simulink model "MotorDriveUnit_TestModel"  (R2025a)
settings: Solver=daessc  StartTime=0.0  StopTime=400  RelTol=1e-3
PreLoadFcn:
  | MotorDriveUnit_TestModelSetup
undefined symbols (not defined in the file or in its folder): batteryHV, Minus, Plus
libraries: fl_lib x22, nesl_utility x10, simulink x5, sdl_lib x1
settings Model: Creator=isaacito  LastModifiedBy=isaacito
settings DataIOCC: DSMLogging=off
settings OptimizationCC: ReuseModelBlockBuffer=off
settings ModelReferenceCC: EnableRefExpFcnMdlSchedulingChecks=on
settings RTWCC: GPUComputeCapability=3.5
settings SimscapeCC: SimscapeLogType=all  SimscapeLogSimulationStatistics=on  SimscapeLogLimitData=off

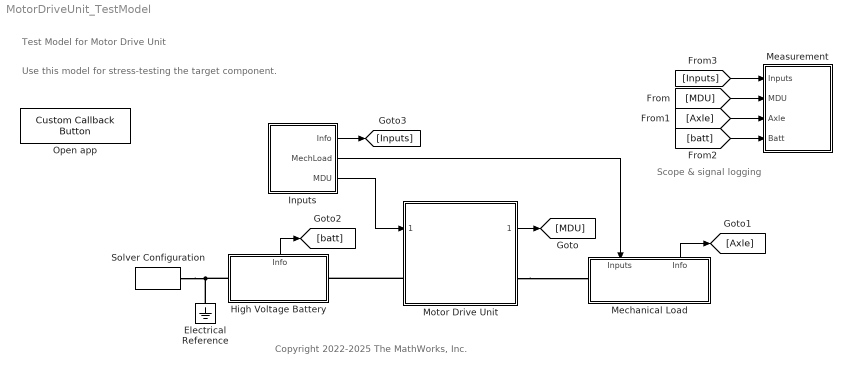
== system MotorDriveUnit_TestModel ==
  note: Test Model for Motor Drive Unit
  note: Copyright 2022-2025 The MathWorks, Inc.
  note: Use this model for stress-testing the target component.
  note: Scope & signal logging
  Electrical Reference : fl_lib/Electrical/Electrical Elements/Electrical Reference
  High Voltage Battery : Subsystem
      settings: PortSchema="{\"entries\":[{\"content\":{\"sides\":[{\"content\":{\"connectorIds\":[\"LConn1\"]},\"type\":\"ConnectorPlacement.EquallySpacedRectSide\",\"uuid\":\"8acd7e9a-bb08-4de6-aa14-0989ebba81b9\"},{\"content\":{\"connectorIds\":[\"RConn1\"],\"side\":\"RIGHT\"},\"type\":\"ConnectorPlacement.EquallySpacedRectSide\",\"uuid\":\"f80e1afc-966f-4d6b-84f9-f0b60dd6f20c\"},{\"content\":{\"connectorIds\":[\"Out1\"],\"side\":\"TOP\"},\"type\":\"ConnectorPlacement.EquallySpacedRectSide\",\"uuid\":\"52ccb2b1-bd5e-4dcb-b9b6-0ef03b912c33\"}]},\"type\":\"ConnectorPlacement.EquallySpacedConnector\",\"uuid\":\"b55f48a4-f283-4a77-8513-99b31abb285a\"}],\"packageUris\":[\"http://schema.mathworks.com/mf0/Connector/R2020b\"],\"version\":\"1.0\"}"
  Inputs : Subsystem
  Measurement : Subsystem
  Mechanical Load : Subsystem
      settings: PortSchema="{\"entries\":[{\"content\":{\"sides\":[{\"content\":{\"connectorIds\":[\"LConn1\"]},\"type\":\"ConnectorPlacement.EquallySpacedRectSide\",\"uuid\":\"18221845-08ef-4cf2-b090-320221152030\"},{\"content\":{\"connectorIds\":[],\"side\":\"RIGHT\"},\"type\":\"ConnectorPlacement.EquallySpacedRectSide\",\"uuid\":\"d5b0548b-74c8-455a-9783-7dc299f3571f\"},{\"content\":{\"connectorIds\":[\"In1\",\"Out1\"],\"side\":\"TOP\"},\"type\":\"ConnectorPlacement.EquallySpacedRectSide\",\"uuid\":\"542d8e55-6d7f-4c9a-9fdc-66897ed9f466\"}]},\"type\":\"ConnectorPlacement.EquallySpacedConnector\",\"uuid\":\"3cd4c536-0337-4305-a842-969bfb1fefe3\"}],\"packageUris\":[\"http://schema.mathworks.com/mf0/Connector/R2020b\"],\"version\":\"1.0\"}"
  Motor Drive Unit : Subsystem  ReferencedSubsystem=MotorDriveUnit_Basic_refsub
      settings: OpenFcn=|
      | % Look under mask:
      | open_system(gcb, "force")
  Open app : CustomCallbackButton  Configuration="{\"components\":[{\"name\":\"BackgroundImageComponent\",\"settings\":{\"image\":{\"size\":[0,0],\"src\":\"default\",\"srcOrientation\":\"Right\"},\"position\":[0,0,1,1]}},{\"name\":\"ButtonStateComponent\",\"settings\":{\"buttonType\":\"momentary\",\"clickFcn\":\"MotorDriveUnitApp\\n\",\"onValue\":1,\"position\":[0,0,1,1],\"pressDelay\":\"500\",\"pressFcn\":\"\",\"repeatInterval\":\"0\",\"states\":[{\"horizontalAlignment\":\"center\",\"image\":{\"position\":[0,0,1,1],\"size\":[1,1],\"src\":\"default\",\"srcOrientation\":\"Right\"},\"label\":{\"color\":[0.01176470588,0.01176470588,0.01176470588,1],\"icon\":{\"size\":[0,0],\"src\":\"default\",\"srcOrientation\":\"Right\"},\"iconOffset\":0,\"iconPlacement\":\"left\",\"opacity\":1,\"show\":true,\"text\":{\"content\":\"Open app\",\"font\":\"Helvetica\"}},\"labelOffset\":[0,0],\"verticalAlignment\":\"middle\"},{\"horizontalAlignment\":\"center\",\"image\":{\"position\":[0,0,1,1],\"size\":[1,1],\"src\":\"default\",\"srcOrientation\":\"Right\"},\"label\":{\"color\":[0.01176470588,0.01176470588,0.01176470588,1],\"icon\":{\"size\":[0,0],\"src\":\"default\",\"srcOrientation\":\"Right\"},\"iconOffset\":0,\"iconPlacement\":\"left\",\"opacity\":1,\"show\":true,\"text\":{\"content\":\"Open app\",\"font\":\"Helvetica\"}},\"labelOffset\":[0,0],\"verticalAlignment\":\"middle\"},{\"horizontalAlignment\":\"center\",\"image\":{\"position\":[0,0,1,1],\"size\":[1,1],\"src\":\"default\",\"srcOrientation\":\"Right\"},\"label\":{\"color\":[0.01176470588,0.01176470588,0.01176470588,1],\"icon\":{\"size\":[0,0],\"src\":\"default\",\"srcOrientation\":\"Right\"},\"iconOffset\":0,\"iconPlacement\":\"left\",\"opacity\":1,\"show\":true,\"text\":{\"content\":\"Open app\",\"font\":\"Helvetica\"}},\"labelOffset\":[0,0],\"verticalAlignment\":\"middle\"},{\"horizontalAlignment\":\"center\",\"image\":{\"position\":[0,0,1,1],\"size\":[1,1],\"src\":\"default\",\"srcOrientation\":\"Right\"},\"label\":{\"color\":[0.01176470588,0.01176470588,0.01176470588,1],\"icon\":{\"size\":[0,0],\"src\":\"default\",\"srcOrientation\":\"Right\"},\"iconOffset\":0,\"iconPlacement\":\"left\",\"opacity\":1,\"show\":true,\"text\":{\"content\":\"Open app\",\"font\":\"Helvetica\"}},\"labelOffset\":[0,0],\"verticalAlignment\":\"middle\"}]}},{\"name\":\"ForegroundImageComponent\",\"settings\":{\"image\":{\"size\":[0,0],\"src\":\"default\",\"srcOrientation\":\"Right\"},\"isForeground\":1,\"position\":[0,0,1,1]}}],\"derived\":{\"blockParameters\":{\"AutoActivate\":true,\"ButtonText\":\"Open app\",\"ButtonType\":\"Momentary\",\"ClickFcn\":\"MotorDriveUnitApp\\n\",\"OnValue\":1,\"PressDelay\":\"500\",\"PressFcn\":\"\",\"RepeatInterval\":\"0\",\"fixedAspectRatio\":\"on\"}},\"settings\":{\"BindingType\":\"standalone\",\"autoActivate\":true,\"backgroundColor\":[244,244,244,1],\"backgroundOffset\":0.2,\"backgroundOpacity\":1,\"fixedAspectRatio\":\"on\",\"foregroundColor\":[0.01176470588,0.01176470588,0.01176470588,1],\"migratedFromLegacy\":true,\"useBackgroundColor\":true,\"variant\":\"callback\",\"version\":\"R2025a\"},\"type\":\"Button\"}"  CustomBackgroundColor="{\"color\":[0.9568627451,0.9568627451,0.9568627451],\"show\":true}"
  Solver Configuration : nesl_utility/Solver Configuration  PhysicalDomain=network_engine_domain  SubClassName=solver  LeftPortType=input  RightPortType=generic  Tones=[]  Harmonics=[]  SimulateNoise=off  Profile=off  UseLocalSampling=off  EnableSwitchedLinearOptims=on  FrequencyDomain=off  UseCCode=off  RelTol=0.001  AbsTol=1e-06  MinStep=1e-09  ToWorkspace=off  RevertToSquareIcSolve=off  NumHomotopyIterations=100  PhasorMode=off  PhasorModeNumHarmonics=1  ConsistencySolver=NEWTON_FTOL  IndexReductionMethod=DerivativeReplacement  DoDC=off  ResidualTolerance=1e-09  ConsistencyTolSource=GLOBAL  ConsistencyAbsTol=0.001  ConsistencyRelTol=0.001  ConsistencyTolFactor=0.001  UseLocalSolver=off  LocalSolverChoice=NE_BACKWARD_EULER_ADVANCER  ResolveIndetEquations=on  FunctionEvalNumThread=1  LocalSolverSampleTime=0.001  DoFixedCost=off  MaxNonlinIter=3  MaxModeIter=2  ComputeImpulses=off  ImpulseIterations=2  LinearAlgebra=auto  LinearAlgebraNumThread=0  EquationFormulation=NE_TIME_EF  DelaysMemoryBudget=1024  AutomaticFiltering=on  FilteringTimeConstant=0.001  PartitionStorageMethod=AS_NEEDED  PartitionMemoryBudget=1024  PartitionMethod=ROBUST  MultibodyUseLocalSolver=off  MultibodyLocalSolverChoice=ODE1  MultibodyLocalSolverSampleTime=0.001
      settings: AttributesFormatString=Local solver %<UseLocalSolver>
  wires:
  Motor Drive Unit/1 -> [MDU]
  [MDU] -> Measurement/2(MDU)
  Inputs/3(MDU) -> Motor Drive Unit/1
  [Axle] -> Measurement/3(Axle)
  High Voltage Battery/1(Info) -> [batt]
  [batt] -> Measurement/4(Batt)
  Inputs/2(MechLoad) -> Mechanical Load/1(Inputs)
  Mechanical Load/1(Info) -> [Axle]
  Inputs/1(Info) -> [Inputs]
  [Inputs] -> Measurement/1(Inputs)
  connections:
  Motor Drive Unit/LConn1 -- High Voltage Battery/RConn1
  Electrical Reference/LConn1 -- High Voltage Battery/LConn1 -- Solver Configuration/RConn1
  Motor Drive Unit/RConn1 -- Mechanical Load/LConn1

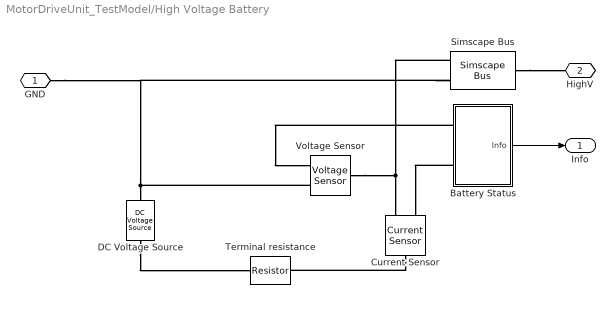
== system MotorDriveUnit_TestModel/High Voltage Battery ==
  Battery Status : Subsystem
  Current Sensor : fl_lib/Electrical/Electrical Sensors/Current Sensor
  DC Voltage Source : fl_lib/Electrical/Electrical Sources/DC Voltage Source  v0=batteryHV.nominalVoltage_V V
      settings: AttributesFormatString=%<v0> [%<v0_unit>]
  Simscape Bus : SimscapeBus  HierarchyStrings=Plus;Minus  ConnectionType=Bus: Bus_HighVoltage
      settings: AttributesFormatString=%<ConnectionType>
  Terminal resistance : fl_lib/Electrical/Electrical Elements/Resistor  R=batteryHV.internalResistance_Ohm Ohm  i_specify=off  i_priority=High  i=0 A  i_nominal_specify=off  i_nominal_value=1  i_nominal_unit=A  v_specify=off  v_priority=High  v=0 V  v_nominal_specify=off  v_nominal_value=1  v_nominal_unit=V
      settings: AttributesFormatString=%<R> [%<R_unit>]
  Voltage Sensor : fl_lib/Electrical/Electrical Sensors/Voltage Sensor
  GND : PMIOPort  Side=Left
  HighV : PMIOPort  Port=2  Side=Right
  Info : Outport
  wires:
  Battery Status/1(Info) -> Info/1
  connections:
  DC Voltage Source/RConn1 -- Simscape Bus/LConn2 -- GND/RConn1 -- Voltage Sensor/RConn2
  Simscape Bus/LConn1 -- Voltage Sensor/LConn1 -- Current Sensor/RConn2
  Battery Status/LConn2 -- Current Sensor/RConn1
  Simscape Bus/RConn1 -- HighV/RConn1
  Current Sensor/LConn1 -- Terminal resistance/RConn1
  DC Voltage Source/LConn1 -- Terminal resistance/LConn1
  Battery Status/LConn1 -- Voltage Sensor/RConn1

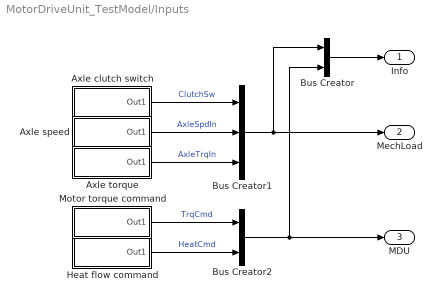
== system MotorDriveUnit_TestModel/Inputs ==
  Axle clutch switch : Subsystem  mask(Piece-Wise Constant Signal){dataPoints=[0 0;1 0]}
      mask prompts: dataPoints "Data points"
      mask help:
      | This block generates a piece-wise constant signal. Data points parameter takes an N-by-2 matrix where each row specifies a constant segment. First column defines the start time of constant segment, and second column specifies the value of it. The value continues until the value of the next segment is defined. The values of the two consecutive rows are connected with a discrete jump.
      |
      | For example, a matrix [0 6; 1 7;2 5] for Data points defines a signal as follows. First row defines a constant segment from t=0 of value 6. Second row defines a point at t=1 of value 7. Third row defines a constant segment from t=2 of value 5. The value makes a discrete jump from one segment to the next.
      mask init:
      | sig = SignalDesigner("PieceWiseConstant");
      | 
      | % Initialization function can access parameter names directly
      | sig.XYData = dataPoints;
      | 
      | update(sig)
      | 
      | SignalSourceBlockCallback.setDataToLookupTableBlock( ...
      |   SignalObject = sig, ...
      |   PathToBlock = [gcb '/1-D Lookup Table']);
      mask DialogControl Control3 Prompt: invisible horizontal spacer 1
      mask DialogControl Control4 Prompt: invisible horizontal spacer 2
      mask DialogControl Control5 Prompt: invisible horizontal spacer 3
      mask DialogControl PlotButton Prompt: Plot
      mask DialogControl PlotButton Callback: SignalSourceBlockCallback.plotPieceWiseConstant(gcb)
      mask Display: disp("Piece-Wise" + newline + "Constant")
  Axle speed : Subsystem  mask(Continuous Multi-Step Signal){dataPoints=[0 1 0], deltaT=10}
      mask prompts: dataPoints "Data points"; deltaT "Interpolation step [s]"
      mask help:
      | This block generates a signal consisting of smoothly connected flat segments. Data points parameter takes an N-by-3 matrix where each row specifies a flat segment. First column and second column define start and end time of the segment, respectively. Third column defines the value of the segment. Second column can also be NaN to define a point value. Flat segments and point values are smoothly interpolated by Akima spline with the specified interpolation step.
      |
      | For example, a matrix [0 1 5; 3 nan 9; 6 8 7] for Data points defines a signal as follows. First row defines a flat segment from t=0 to t=1 of value 5. Second row defines a point at t=3 of value 9. Third row defines a flat segment from t=6 to t=8 of value 7.
      mask init:
      | sig = SignalDesigner("ContinuousMultiStep");
      | 
      | % Initialization function can access parameter names directly
      | sig.XYData = dataPoints;
      | sig.DeltaX = deltaT;
      | 
      | update(sig)
      | 
      | SignalSourceBlockCallback.setDataToLookupTableBlock( ...
      |   SignalObject = sig, ...
      |   PathToBlock = [gcb '/1-D Lookup Table']);
      mask DialogControl Control3 Prompt: horizontal spacer 1
      mask DialogControl Control4 Prompt: horizontal spacer 2
      mask DialogControl Control5 Prompt: horizontal spacer 3
      mask DialogControl PlotButton Prompt: Plot
      mask DialogControl PlotButton Callback: SignalSourceBlockCallback.plotContinuousMultiStep(gcb);
      mask Display: disp("Continuous" + newline + "Multi-Step")
  Axle torque : Subsystem  mask(Continuous Multi-Step Signal){dataPoints=[0 20 0;21 300 -10], deltaT=0.1}
      mask prompts: dataPoints "Data points"; deltaT "Interpolation step [s]"
      mask help:
      | This block generates a signal consisting of smoothly connected flat segments. Data points parameter takes an N-by-3 matrix where each row specifies a flat segment. First column and second column define start and end time of the segment, respectively. Third column defines the value of the segment. Second column can also be NaN to define a point value. Flat segments and point values are smoothly interpolated by Akima spline with the specified interpolation step.
      |
      | For example, a matrix [0 1 5; 3 nan 9; 6 8 7] for Data points defines a signal as follows. First row defines a flat segment from t=0 to t=1 of value 5. Second row defines a point at t=3 of value 9. Third row defines a flat segment from t=6 to t=8 of value 7.
      mask init: same as MotorDriveUnit_TestModel/Inputs/Axle speed
      mask DialogControl Control3 Prompt: horizontal spacer 1
      mask DialogControl Control4 Prompt: horizontal spacer 2
      mask DialogControl Control5 Prompt: horizontal spacer 3
      mask DialogControl PlotButton Prompt: Plot
      mask DialogControl PlotButton Callback: SignalSourceBlockCallback.plotContinuousMultiStep(gcb);
      mask Display: disp("Continuous" + newline + "Multi-Step")
  Bus Creator : BusCreator  Inputs=2
  Bus Creator1 : BusCreator  Inputs=3
  Bus Creator2 : BusCreator  Inputs=2
  Heat flow command : Subsystem  mask(Continuous Multi-Step Signal){dataPoints=[0 50 0;60 200 -2000;250 300 -12000], deltaT=1}
      mask prompts: dataPoints "Data points"; deltaT "Interpolation step [s]"
      mask help:
      | This block generates a signal consisting of smoothly connected flat segments. Data points parameter takes an N-by-3 matrix where each row specifies a flat segment. First column and second column define start and end time of the segment, respectively. Third column defines the value of the segment. Second column can also be NaN to define a point value. Flat segments and point values are smoothly interpolated by Akima spline with the specified interpolation step.
      |
      | For example, a matrix [0 1 5; 3 nan 9; 6 8 7] for Data points defines a signal as follows. First row defines a flat segment from t=0 to t=1 of value 5. Second row defines a point at t=3 of value 9. Third row defines a flat segment from t=6 to t=8 of value 7.
      mask init: same as MotorDriveUnit_TestModel/Inputs/Axle speed
      mask DialogControl Control3 Prompt: horizontal spacer 1
      mask DialogControl Control4 Prompt: horizontal spacer 2
      mask DialogControl Control5 Prompt: horizontal spacer 3
      mask DialogControl PlotButton Prompt: Plot
      mask DialogControl PlotButton Callback: SignalSourceBlockCallback.plotContinuousMultiStep(gcb);
      mask Display: disp("Continuous" + newline + "Multi-Step")
  Motor torque command : Subsystem  mask(Continuous Multi-Step Signal){dataPoints=[0 10 0;60 100 -300;105 200 200;205 300 250], deltaT=0.5}
      mask prompts: dataPoints "Data points"; deltaT "Interpolation step [s]"
      mask help:
      | This block generates a signal consisting of smoothly connected flat segments. Data points parameter takes an N-by-3 matrix where each row specifies a flat segment. First column and second column define start and end time of the segment, respectively. Third column defines the value of the segment. Second column can also be NaN to define a point value. Flat segments and point values are smoothly interpolated by Akima spline with the specified interpolation step.
      |
      | For example, a matrix [0 1 5; 3 nan 9; 6 8 7] for Data points defines a signal as follows. First row defines a flat segment from t=0 to t=1 of value 5. Second row defines a point at t=3 of value 9. Third row defines a flat segment from t=6 to t=8 of value 7.
      mask init: same as MotorDriveUnit_TestModel/Inputs/Axle speed
      mask DialogControl Control3 Prompt: horizontal spacer 1
      mask DialogControl Control4 Prompt: horizontal spacer 2
      mask DialogControl Control5 Prompt: horizontal spacer 3
      mask DialogControl PlotButton Prompt: Plot
      mask DialogControl PlotButton Callback: SignalSourceBlockCallback.plotContinuousMultiStep(gcb);
      mask Display: disp("Continuous" + newline + "Multi-Step")
  Info : Outport
  MechLoad : Outport  Port=2
  MDU : Outport  Port=3
  wires:
  Bus Creator/1 -> Info/1
  Motor torque command/1(Out1) -> Bus Creator2/1  "TrqCmd"
  Axle torque/1(Out1) -> Bus Creator1/3  "AxleTrqIn"
  Axle speed/1(Out1) -> Bus Creator1/2  "AxleSpdIn"
  Axle clutch switch/1(Out1) -> Bus Creator1/1  "ClutchSw"
  Bus Creator1/1 -> Bus Creator/1, MechLoad/1
  Bus Creator2/1 -> Bus Creator/2, MDU/1
  Heat flow command/1(Out1) -> Bus Creator2/2  "HeatCmd"

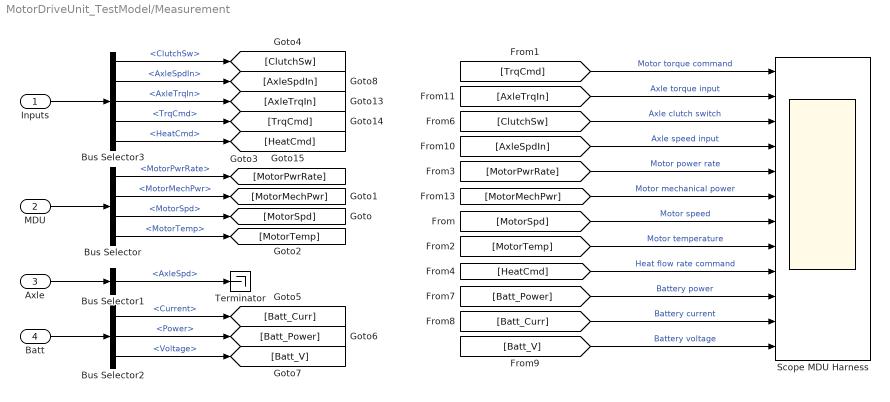
== system MotorDriveUnit_TestModel/Measurement ==
  Inputs : Inport
  MDU : Inport  Port=2
  Axle : Inport  Port=3
  Batt : Inport  Port=4
  Bus Selector : BusSelector  OutputSignals=MotorPwrRate,MotorMechPwr,MotorSpd,MotorTemp
  Bus Selector1 : BusSelector  OutputSignals=AxleSpd
  Bus Selector2 : BusSelector  OutputSignals=Current,Power,Voltage
  Bus Selector3 : BusSelector  OutputSignals=signal1.ClutchSw,signal1.AxleSpdIn,signal1.AxleTrqIn,signal2.TrqCmd,signal2.HeatCmd
  Scope MDU Harness : Scope  NumInputPorts=12
      settings: ActiveDisplayYMinimum=-368.75  ActiveDisplayYMaximum=318.75
  Terminator : Terminator
  wires:
  MDU/1 -> Bus Selector/1
  Bus Selector/3 -> [MotorSpd]  "<MotorSpd>"
  Bus Selector/4 -> [MotorTemp]  "<MotorTemp>"
  Axle/1 -> Bus Selector1/1
  Bus Selector2/3 -> [Batt_V]  "<Voltage>"
  Bus Selector2/2 -> [Batt_Power]  "<Power>"
  Bus Selector2/1 -> [Batt_Curr]  "<Current>"
  Batt/1 -> Bus Selector2/1
  Bus Selector1/1 -> Terminator/1  "<AxleSpd>"
  Bus Selector/1 -> [MotorPwrRate]  "<MotorPwrRate>"
  Inputs/1 -> Bus Selector3/1
  Bus Selector3/1 -> [ClutchSw]  "<ClutchSw>"
  Bus Selector3/2 -> [AxleSpdIn]  "<AxleSpdIn>"
  Bus Selector3/3 -> [AxleTrqIn]  "<AxleTrqIn>"
  Bus Selector3/4 -> [TrqCmd]  "<TrqCmd>"
  Bus Selector3/5 -> [HeatCmd]  "<HeatCmd>"
  Bus Selector/2 -> [MotorMechPwr]  "<MotorMechPwr>"
  [MotorPwrRate] -> Scope MDU Harness/5  "Motor power rate"
  [TrqCmd] -> Scope MDU Harness/1  "Motor torque command"
  [MotorMechPwr] -> Scope MDU Harness/6  "Motor mechanical power"
  [MotorSpd] -> Scope MDU Harness/7  "Motor speed"
  [MotorTemp] -> Scope MDU Harness/8  "Motor temperature"
  [HeatCmd] -> Scope MDU Harness/9  "Heat flow rate command"
  [Batt_Power] -> Scope MDU Harness/10  "Battery power"
  [Batt_Curr] -> Scope MDU Harness/11  "Battery current"
  [Batt_V] -> Scope MDU Harness/12  "Battery voltage"
  [AxleTrqIn] -> Scope MDU Harness/2  "Axle torque input"
  [ClutchSw] -> Scope MDU Harness/3  "Axle clutch switch"
  [AxleSpdIn] -> Scope MDU Harness/4  "Axle speed input"

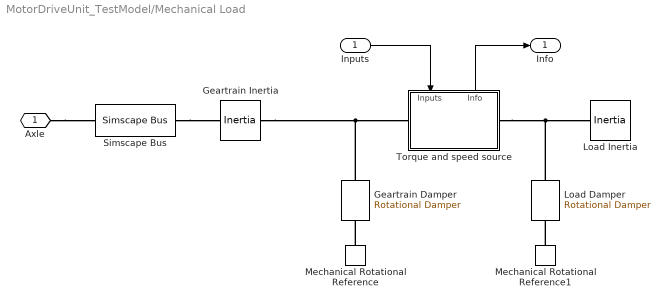
== system MotorDriveUnit_TestModel/Mechanical Load ==
  Inputs : Inport
  Geartrain Damper : fl_lib/Mechanical/Rotational Elements/Rotational Damper  D=0.001 m*N/rpm  w_specify=off  w_priority=None  w=0 rad/s  w_nominal_specify=off  w_nominal_value=1  w_nominal_unit=rad/s  t_specify=off  t_priority=None  t=0 N*m  t_nominal_specify=off  t_nominal_value=1  t_nominal_unit=N*m
      settings: AttributesFormatString=|
      | %<D>
      | %<D_unit>
  Geartrain Inertia : fl_lib/Mechanical/Rotational Elements/Inertia  inertia=1.35 kg*m^2  num_ports=foundation.enum.numPorts2.two  w_specify=on  w_priority=None  w=0 rpm  w_nominal_specify=off  w_nominal_value=1  w_nominal_unit=rad/s  t_specify=off  t_priority=None  t=0 N*m  t_nominal_specify=off  t_nominal_value=1  t_nominal_unit=N*m
      settings: InternalSimscapePortConfiguration="{\"Bottom\":[],\"Left\":[{\"id\":\"I\",\"label\":\"\",\"type\":\"foundation.mechanical.rotational.rotational\"}],\"Right\":[{\"id\":\"J\",\"label\":\"\",\"type\":\"foundation.mechanical.rotational.rotational\"}],\"Top\":[]}"
      settings: AttributesFormatString=|
      | %<inertia> %<inertia_unit>
      | Priority: %<w_priority>
  Load Damper : fl_lib/Mechanical/Rotational Elements/Rotational Damper  D=0.03 N*m/rpm  w_specify=off  w_priority=None  w=0 rad/s  w_nominal_specify=off  w_nominal_value=1  w_nominal_unit=rad/s  t_specify=off  t_priority=None  t=0 N*m  t_nominal_specify=off  t_nominal_value=1  t_nominal_unit=N*m
      settings: AttributesFormatString=|
      | %<D>
      | %<D_unit>
  Load Inertia : fl_lib/Mechanical/Rotational Elements/Inertia  inertia=9 kg*m^2  num_ports=foundation.enum.numPorts2.one  w_specify=on  w_priority=High  w=initial.loadInertiaSpd_rpm rpm  w_nominal_specify=off  w_nominal_value=1  w_nominal_unit=rad/s  t_specify=off  t_priority=None  t=0 N*m  t_nominal_specify=off  t_nominal_value=1  t_nominal_unit=N*m
      settings: AttributesFormatString=|
      | %<inertia> [%<inertia_unit>]
      | %<w> [%<w_unit>]
      | Priority: %<w_priority>
  Mechanical Rotational Reference : fl_lib/Mechanical/Rotational Elements/Mechanical Rotational Reference
  Mechanical Rotational Reference1 : fl_lib/Mechanical/Rotational Elements/Mechanical Rotational Reference
  Simscape Bus : SimscapeBus  HierarchyStrings=AngSpd  ConnectionType=Bus: Bus_Rotational
  Torque and speed source : Subsystem
      settings: PortSchema="{\"entries\":[{\"content\":{\"sides\":[{\"content\":{\"connectorIds\":[\"LConn1\"]},\"type\":\"ConnectorPlacement.EquallySpacedRectSide\",\"uuid\":\"92a06674-aaa2-495f-b380-fd1e5a218eb3\"},{\"content\":{\"connectorIds\":[\"RConn1\"],\"side\":\"RIGHT\"},\"type\":\"ConnectorPlacement.EquallySpacedRectSide\",\"uuid\":\"3e9807eb-b215-4ab1-ac02-6574a58f93c0\"},{\"content\":{\"connectorIds\":[\"In1\",\"Out1\"],\"side\":\"TOP\"},\"type\":\"ConnectorPlacement.EquallySpacedRectSide\",\"uuid\":\"937668c8-63b6-43a7-85c7-81bf7d359316\"}]},\"type\":\"ConnectorPlacement.EquallySpacedConnector\",\"uuid\":\"ba9b6e46-9639-4838-8d50-8636a64d3a24\"}],\"packageUris\":[\"http://schema.mathworks.com/mf0/Connector/R2020b\"],\"version\":\"1.0\"}"
  Axle : PMIOPort  Side=Left
  Info : Outport
  wires:
  Torque and speed source/1(Info) -> Info/1
  Inputs/1 -> Torque and speed source/1(Inputs)
  connections:
  Mechanical Rotational Reference/LConn1 -- Geartrain Damper/RConn1
  Mechanical Rotational Reference1/LConn1 -- Load Damper/RConn1
  Simscape Bus/LConn1 -- Geartrain Inertia/RConn1
  Axle/RConn1 -- Simscape Bus/RConn1
  Torque and speed source/RConn1 -- Load Damper/LConn1 -- Load Inertia/LConn1
  Geartrain Inertia/LConn1 -- Geartrain Damper/LConn1 -- Torque and speed source/LConn1

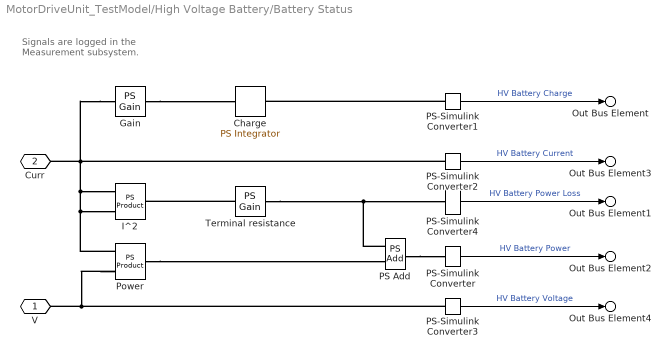
== system MotorDriveUnit_TestModel/High Voltage Battery/Battery Status ==
  note: Signals are logged in
      | the Measurement subsystem.
  Charge : fl_lib/Physical Signals/Linear Operators/PS Integrator  reset_method=foundation.enum.IntegratorResetSpec.None  initial_condition_spec=foundation.enum.IntegratorICSpec.Internal  saturation_spec=foundation.enum.IntegratorSaturationSpec.None  saturation_source_spec=foundation.enum.IntegratorSaturationSourceSpec.Internal  x0=0 A*hr  xu=inf s  xl=-inf s
      settings: AttributesFormatString=%<x0> [%<x0_unit>]
  Gain : fl_lib/Physical Signals/Functions/PS Gain  gain=-1
      settings: AttributesFormatString=%<gain>
  I^2 : fl_lib/Physical Signals/Functions/PS Product
  PS Add : fl_lib/Physical Signals/Functions/PS Add
  PS-Simulink Converter : nesl_utility/PS-Simulink Converter  PhysicalDomain=network_engine_domain  SubClassName=ps_output  LeftPortType=input  RightPortType=output  PseudoPeriodic=off  Frequencies=[]  VectorFormat=1-D array  Unit=kW  AffineConversion=off
  PS-Simulink Converter1 : nesl_utility/PS-Simulink Converter  PhysicalDomain=network_engine_domain  SubClassName=ps_output  LeftPortType=input  RightPortType=output  PseudoPeriodic=off  Frequencies=[]  VectorFormat=1-D array  Unit=A*hr  AffineConversion=off
  PS-Simulink Converter2 : nesl_utility/PS-Simulink Converter  PhysicalDomain=network_engine_domain  SubClassName=ps_output  LeftPortType=input  RightPortType=output  PseudoPeriodic=off  Frequencies=[]  VectorFormat=1-D array  Unit=A  AffineConversion=off
  PS-Simulink Converter3 : nesl_utility/PS-Simulink Converter  PhysicalDomain=network_engine_domain  SubClassName=ps_output  LeftPortType=input  RightPortType=output  PseudoPeriodic=off  Frequencies=[]  VectorFormat=1-D array  Unit=V  AffineConversion=off
  PS-Simulink Converter4 : nesl_utility/PS-Simulink Converter  PhysicalDomain=network_engine_domain  SubClassName=ps_output  LeftPortType=input  RightPortType=output  PseudoPeriodic=off  Frequencies=[]  VectorFormat=1-D array  Unit=W  AffineConversion=off
  Power : fl_lib/Physical Signals/Functions/PS Product
  Terminal resistance : fl_lib/Physical Signals/Functions/PS Gain  gain=batteryHV.internalResistance_Ohm Ohm
      settings: AttributesFormatString=%<gain> [%<gain_unit>]
  V : PMIOPort  Side=Left
  Curr : PMIOPort  Port=2  Side=Left
  Out Bus Element : Outport  PortName=Info  Element=Charge
      settings: AttributesFormatString=%<Unit>
  Out Bus Element3 : Outport  PortName=Info  Element=Current
      settings: AttributesFormatString=%<Unit>
  Out Bus Element1 : Outport  PortName=Info  Element=PowerLoss
      settings: AttributesFormatString=%<Unit>
  Out Bus Element2 : Outport  PortName=Info  Element=Power
      settings: AttributesFormatString=%<Unit>
  Out Bus Element4 : Outport  PortName=Info  Element=Voltage
      settings: AttributesFormatString=%<Unit>
  wires:
  PS-Simulink Converter3/1 -> Out Bus Element4/1  "HV Battery Voltage"
  PS-Simulink Converter2/1 -> Out Bus Element3/1  "HV Battery Current"
  PS-Simulink Converter4/1 -> Out Bus Element1/1  "HV Battery Power Loss"
  PS-Simulink Converter1/1 -> Out Bus Element/1  "HV Battery Charge"
  PS-Simulink Converter/1 -> Out Bus Element2/1  "HV Battery Power"
  connections:
  Power/RConn1 -- PS Add/LConn2
  PS Add/RConn1 -- PS-Simulink Converter/LConn1
  Terminal resistance/LConn1 -- I^2/RConn1
  PS-Simulink Converter1/LConn1 -- Charge/RConn1
  Gain/RConn1 -- Charge/LConn1
  PS Add/LConn1 -- Terminal resistance/RConn1 -- PS-Simulink Converter4/LConn1
  Power/LConn1 -- V/RConn1 -- PS-Simulink Converter3/LConn1
  Gain/LConn1 -- PS-Simulink Converter2/LConn1 -- Curr/RConn1 -- I^2/LConn1 -- Power/LConn2 -- I^2/LConn2

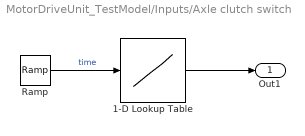
== system MotorDriveUnit_TestModel/Inputs/Axle clutch switch ==
  1-D Lookup Table : Lookup_n-D  NumberOfTableDimensions=1  BreakpointsForDimension1="[0  1]"  Table="[0  0]"  InterpMethod=Flat  InternalRulePriority=Speed  RndMeth=Simplest
  Ramp : simulink/Sources/Ramp  slope=1  start=0  InitialOutput=0
      settings: AttributesFormatString=|
      | Slope: %<slope>
      | Start time: %<start>
      | Initial output: %<InitialOutput>
  Out1 : Outport
  wires:
  Ramp/1 -> 1-D Lookup Table/1  "time"
  1-D Lookup Table/1 -> Out1/1

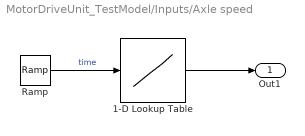
== system MotorDriveUnit_TestModel/Inputs/Axle speed ==
  1-D Lookup Table : Lookup_n-D  NumberOfTableDimensions=1  BreakpointsForDimension1="[0  1]"  Table="[0  0]"  InternalRulePriority=Speed  RndMeth=Simplest
  Ramp : simulink/Sources/Ramp  slope=1  start=0  InitialOutput=0
      settings: AttributesFormatString=|
      | Slope: %<slope>
      | Start time: %<start>
      | Initial output: %<InitialOutput>
  Out1 : Outport
  wires:
  1-D Lookup Table/1 -> Out1/1
  Ramp/1 -> 1-D Lookup Table/1  "time"

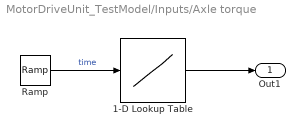
== system MotorDriveUnit_TestModel/Inputs/Axle torque ==
  1-D Lookup Table : Lookup_n-D  NumberOfTableDimensions=1  BreakpointsForDimension1="[0            20          20.1          20.2          20.3          20.4          20.5          20.6          20.7          20.8          20.9            21           300]"  Table="[0            0        -0.28        -1.04        -2.16        -3.52           -5        -6.48        -7.84        -8.96        -9.72          -10          -10]"  InternalRulePriority=Speed  RndMeth=Simplest
  Ramp : simulink/Sources/Ramp  slope=1  start=0  InitialOutput=0
      settings: AttributesFormatString=|
      | Slope: %<slope>
      | Start time: %<start>
      | Initial output: %<InitialOutput>
  Out1 : Outport
  wires:
  Ramp/1 -> 1-D Lookup Table/1  "time"
  1-D Lookup Table/1 -> Out1/1

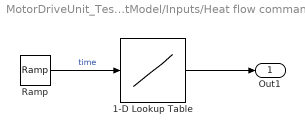
== system MotorDriveUnit_TestModel/Inputs/Heat flow command ==
  1-D Lookup Table : Lookup_n-D  NumberOfTableDimensions=1  BreakpointsForDimension1="[0   50   51   52   53   54   55   56   57   58   59   60  200  201  202  203  204  205  206  207  208  209  210  211  212  213  214  215  216  217  218  219  220  221  222  223  224  225  226  227  228  229  230  231  232  233  234  235  236  237  238  239  240  241  242  243  244  245  246  247  248  249  250  300]"  Table="[0               0             -56            -208            -432            -704           -1000           -1296           -1568           -1792           -1944           -2000           -2000        -2011.84        -2046.72        -2103.68        -2181.76           -2280        -2397.44        -2533.12        -2686.08        -2855.36           -3040        -3239.04        -3451.52        -3676.48        -3912.96           -4160        -4416.64        -4681.92        -4954.88        -5234.56           -5520        -5810.24        -6104.32        -6401.28        -6700.16           -7000        -7299.84        -7598.72        -7895.68        -8189.76           -8480        -8765.44        -9045.12        -9318.08        -9583.36           -9840       -10087.04       -10323.52       -10548.48       -10760.96          -10960       -11144.64       -11313.92       -11466.88       -11602.56          -11720       -11818.24       -11896.32       -11953.28       -11988.16          -12000          -12000]"  InternalRulePriority=Speed  RndMeth=Simplest
  Ramp : simulink/Sources/Ramp  slope=1  start=0  InitialOutput=0
      settings: AttributesFormatString=|
      | Slope: %<slope>
      | Start time: %<start>
      | Initial output: %<InitialOutput>
  Out1 : Outport
  wires:
  Ramp/1 -> 1-D Lookup Table/1  "time"
  1-D Lookup Table/1 -> Out1/1

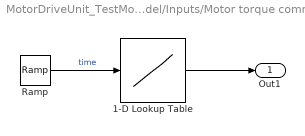
== system MotorDriveUnit_TestModel/Inputs/Motor torque command ==
  1-D Lookup Table : Lookup_n-D  NumberOfTableDimensions=1  BreakpointsForDimension1="[0            10          10.5            11          11.5            12          12.5            13          13.5            14          14.5            15          15.5            16          16.5            17          17.5            18          18.5            19          19.5            20          20.5            21          21.5            22          22.5            23          23.5            24          24.5            25          25.5            26          26.5            27          27.5            28          28.5            29          29.5            30          30.5            31          31.5            32          32.5            33          33.5            34          34.5            35          35.5            36          36.5            37          37.5            38          38.5            39          39.5            40          40.5            41          41.5            42          42.5            43          43.5            44          44.5            45          45.5            46          46.5            47          47.5            48          48.5            49          49.5            50          50.5            51          51.5            52          52.5            53          53.5            54          54.5            55          55.5            56          56.5            57          57.5            58          58.5            59          59.5            60           100         100.5           101         101.5           102         102.5           103         103.5           104         104.5           105           200         200.5           201         201.5           202         202.5           203         203.5           204         204.5           205           300]"  Table="[0             0       -0.0894       -0.3552       -0.7938       -1.4016        -2.175       -3.1104       -4.2042       -5.4528       -6.8526          -8.4      -10.0914      -11.9232      -13.8918      -15.9936       -18.225      -20.5824      -23.0622      -25.6608      -28.3746         -31.2      -34.1334      -37.1712      -40.3098      -43.5456       -46.875      -50.2944      -53.8002      -57.3888      -61.0566         -64.8      -68.6154      -72.4992      -76.4478      -80.4576       -84.525      -88.6464      -92.8182      -97.0368     -101.2986        -105.6     -109.9374     -114.3072     -118.7058     -123.1296      -127.575     -132.0384     -136.5162     -141.0048     -145.5006          -150     -154.4994     -158.9952     -163.4838     -167.9616      -172.425     -176.8704     -181.2942     -185.6928     -190.0626        -194.4     -198.7014     -202.9632     -207.1818     -211.3536      -215.475     -219.5424     -223.5522     -227.5008     -231.3846        -235.2     -238.9434     -242.6112     -246.1998     -249.7056      -253.125     -256.4544     -259.6902     -262.8288     -265.8666        -268.8     -271.6254     -274.3392     -276.9378     -279.4176      -281.775     -284.0064     -286.1082     -288.0768     -289.9086        -291.6     -293.1474     -294.5472     -295.7958     -296.8896      -297.825     -298.5984     -299.2062     -299.6448     -299.9106          -300          -300          -286          -248          -192          -124           -50            24            92           148           186           200           200         201.4         205.2         210.8         217.6           225         232.4         239.2         244.8         248.6           250           250]"  InternalRulePriority=Speed  RndMeth=Simplest
  Ramp : simulink/Sources/Ramp  slope=1  start=0  InitialOutput=0
      settings: AttributesFormatString=|
      | Slope: %<slope>
      | Start time: %<start>
      | Initial output: %<InitialOutput>
  Out1 : Outport
  wires:
  1-D Lookup Table/1 -> Out1/1
  Ramp/1 -> 1-D Lookup Table/1  "time"

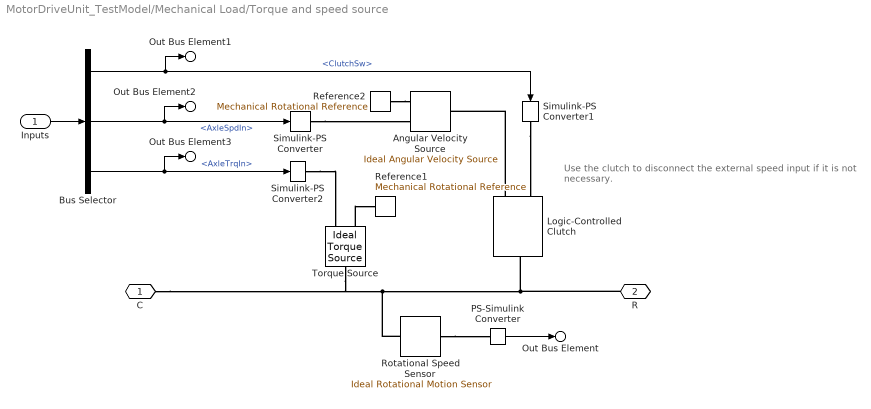
== system MotorDriveUnit_TestModel/Mechanical Load/Torque and speed source ==
  note: Use the clutch to disconnect the external speed input if it is not necessary.
  Inputs : Inport
  Angular Velocity Source : fl_lib/Mechanical/Mechanical Sources/Ideal Angular Velocity Source
  Bus Selector : BusSelector  OutputSignals=ClutchSw,AxleSpdIn,AxleTrqIn
  Logic-Controlled Clutch : sdl_lib/Clutches/Logic-Controlled Clutch  transition_model=sdl.enum.transitionModel.instant  transition_time_constant=0.1 s  t_friction=5000 N*m  t_locked=5000 N*m  w_tol=0.1 rpm  initial_state_locked=sdl.enum.initial_lock.unlocked
      settings: InternalSimscapePortConfiguration="{\"Bottom\":[],\"Left\":[{\"id\":\"E\",\"label\":\"E\",\"type\":\"input\"},{\"id\":\"B\",\"label\":\"B\",\"type\":\"foundation.mechanical.rotational.rotational\"}],\"Right\":[{\"id\":\"F\",\"label\":\"F\",\"type\":\"foundation.mechanical.rotational.rotational\"}],\"Top\":[]}"
  PS-Simulink Converter : nesl_utility/PS-Simulink Converter  PhysicalDomain=network_engine_domain  SubClassName=ps_output  LeftPortType=input  RightPortType=output  PseudoPeriodic=off  Frequencies=[]  VectorFormat=inherit  Unit=rpm  AffineConversion=off
  Reference1 : fl_lib/Mechanical/Rotational Elements/Mechanical Rotational Reference
  Reference2 : fl_lib/Mechanical/Rotational Elements/Mechanical Rotational Reference
  Rotational Speed Sensor : fl_lib/Mechanical/Mechanical Sensors/Ideal Rotational Motion Sensor  reference=foundation.enum.MeasurementReference.absolute  acceleration_port=false  velocity_port=true  position_port=false  wrap_angle=simscape.enum.onoff.off  offset=0 rad
      settings: InternalSimscapePortConfiguration="{\"Bottom\":[],\"Left\":[{\"id\":\"R\",\"label\":\"R\",\"type\":\"foundation.mechanical.rotational.rotational\"}],\"Right\":[{\"id\":\"W\",\"label\":\"W\",\"type\":\"output\"}],\"Top\":[]}"
  Simulink-PS Converter : nesl_utility/Simulink-PS Converter  PhysicalDomain=network_engine_domain  SubClassName=ps_input  LeftPortType=input  RightPortType=output  PseudoPeriodic=off  Frequencies=[]  NoiseDistribution=none  NoiseParameters=[]  Unit=rpm  AffineConversion=off  FilteringAndDerivatives=filter  SimscapeFilterOrder=1  InputFilterTimeConstant=0.001  UdotUserProvided=1
  Simulink-PS Converter2 : nesl_utility/Simulink-PS Converter  PhysicalDomain=network_engine_domain  SubClassName=ps_input  LeftPortType=input  RightPortType=output  PseudoPeriodic=off  Frequencies=[]  NoiseDistribution=none  NoiseParameters=[]  Unit=N*m  AffineConversion=off  FilteringAndDerivatives=filter  SimscapeFilterOrder=1  InputFilterTimeConstant=0.001  UdotUserProvided=1
  Simulink-PS Converter1 : nesl_utility/Simulink-PS Converter  PhysicalDomain=network_engine_domain  SubClassName=ps_input  LeftPortType=input  RightPortType=output  PseudoPeriodic=off  Frequencies=[]  NoiseDistribution=none  NoiseParameters=[]  Unit=1  AffineConversion=off  FilteringAndDerivatives=provide  SimscapeFilterOrder=1  InputFilterTimeConstant=0.001  UdotUserProvided=0
      settings: AttributesFormatString=|
      | %<Unit>
      | Derivative: %<FilteringAndDerivatives>
  Torque Source : fl_lib/Mechanical/Mechanical Sources/Ideal Torque Source
  C : PMIOPort  Side=Left
  R : PMIOPort  Port=2  Side=Right
  Out Bus Element : Outport  PortName=Info  Element=AxleSpd
  Out Bus Element1 : Outport  PortName=Info  Element=AxleClutchSw
  Out Bus Element2 : Outport  PortName=Info  Element=AxleSpdIn
  Out Bus Element3 : Outport  PortName=Info  Element=AxleTrqIn
  wires:
  Inputs/1 -> Bus Selector/1
  Bus Selector/1 -> Out Bus Element1/1, Simulink-PS Converter1/1  "<ClutchSw>"
  Bus Selector/2 -> Simulink-PS Converter/1, Out Bus Element2/1  "<AxleSpdIn>"
  Bus Selector/3 -> Out Bus Element3/1, Simulink-PS Converter2/1  "<AxleTrqIn>"
  PS-Simulink Converter/1 -> Out Bus Element/1
  connections:
  Simulink-PS Converter/RConn1 -- Angular Velocity Source/RConn1
  Reference2/LConn1 -- Angular Velocity Source/RConn2
  Logic-Controlled Clutch/LConn2 -- Angular Velocity Source/LConn1
  Simulink-PS Converter1/RConn1 -- Logic-Controlled Clutch/LConn1
  Rotational Speed Sensor/LConn1 -- C/RConn1 -- Torque Source/LConn1 -- R/RConn1 -- Logic-Controlled Clutch/RConn1
  Rotational Speed Sensor/RConn1 -- PS-Simulink Converter/LConn1
  Simulink-PS Converter2/RConn1 -- Torque Source/RConn1
  Torque Source/RConn2 -- Reference1/LConn1
